simulink model "Is_pos_def"  (Simulink 8.1)
settings: Solver=ode45  StartTime=0.0  StopTime=10.0  RelTol=1e-3
libraries: simulink x1
settings Model: Creator=dejanira  LastModifiedBy=dejanira
settings DataIOCC: SignalLoggingSaveFormat=Dataset
settings OptimizationCC: ExpressionDepthLimit=128
settings DebuggingCC: FcnCallInpInsideContextMsg=EnableAllAsError
settings GRTTargetCC: CombineOutputUpdateFcns=on  GRTInterface=off

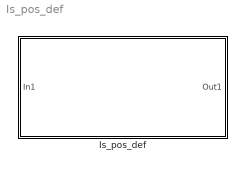
== system Is_pos_def ==
  Is_pos_def : Subsystem  TreatAsAtomicUnit=on  mask(Is_pos_def){}
      mask Display:
      | port_label('input',1,'matrix')
      | port_label('output',1,'T/F')

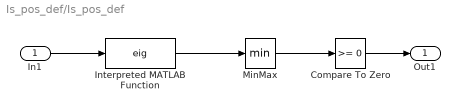
== system Is_pos_def/Is_pos_def ==
  In1 : Inport
  Compare To Zero : simulink/Logic and Bit Operations/Compare To Zero  relop=>=  OutDataTypeStr=boolean
  Interpreted MATLAB Function : MATLABFcn  MATLABFcn=eig
  MinMax : MinMax
  Out1 : Outport
  wires:
  MinMax/1 -> Compare To Zero/1
  In1/1 -> Interpreted MATLAB Function/1
  Compare To Zero/1 -> Out1/1
  Interpreted MATLAB Function/1 -> MinMax/1
